simulink model "SanityCheckZ"  (R2023a)
settings: Solver=VariableStepAuto  StartTime=0.0  StopTime=10.0  RelTol=1e-3
settings Model: Creator=aan18022  LastModifiedBy=asd19005

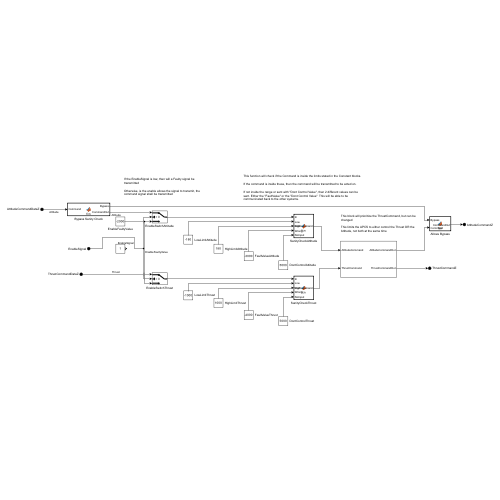
[thumbnail: Simulink's stored preview of the top-level diagram]
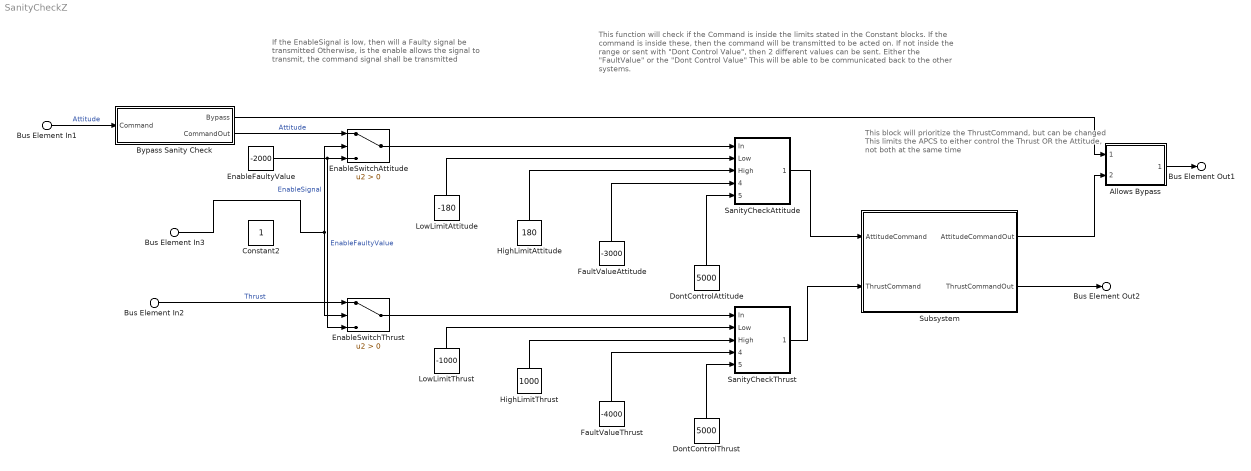
== system SanityCheckZ ==
  note: If the EnableSignal is low, then will a Faulty signal be transmitted
      |
      | Otherwise, is the enable allows the signal to transmit, the command signal shall be transmitted
  note: This function will check if the Command is inside the limits stated in the Constant blocks.
      |
      | If the command is inside these, then the command will be transmitted to be acted on.
      |
      | If not inside the range or sent with "Dont Control Value", then 2 different values can be sent. Either the "FaultValue" or the "Dont Control Value"  This will be able to be communicated back to the other systems.
  note: This block will prioritize the ThrustCommand, but can be changed
      |
      | This limits the APCS to either control the Thrust OR the Attitude, not both at the same time
  Bus Element In3 : Inport  PortName=EnableSignal
  Bus Element In1 : Inport  Port=2  PortName=AttitudeCommandDataZ
  Bus Element In2 : Inport  Port=3  PortName=ThrustCommandDataZ
  Allows Bypass : MATLAB Function  TreatAsAtomicUnit=on
  Bypass Sanity Check : MATLAB Function  TreatAsAtomicUnit=on
  Constant2 : Constant
  DontControlAttitude : Constant  Value=5000
  DontControlThrust : Constant  Value=5000
  EnableFaultyValue : Constant  Value=-2000
  EnableSwitchAttitude : Switch  Criteria=u2 > Threshold  SaturateOnIntegerOverflow=off  InputSameDT=off
  EnableSwitchThrust : Switch  Criteria=u2 > Threshold  SaturateOnIntegerOverflow=off  InputSameDT=off
  FaultValueAttitude : Constant  Value=-3000
  FaultValueThrust : Constant  Value=-4000
  HighLimitAttitude : Constant  Value=180
  HighLimitThrust : Constant  Value=1000
  LowLimitAttitude : Constant  Value=-180
  LowLimitThrust : Constant  Value=-1000
  SanityCheckAttitude : MATLAB Function  TreatAsAtomicUnit=on
  SanityCheckThrust : MATLAB Function  TreatAsAtomicUnit=on
  Subsystem : Subsystem
  Bus Element Out1 : Outport  PortName=AttitudeCommandZ
  Bus Element Out2 : Outport  Port=2  PortName=ThrustCommandZ
  wires:
  EnableSwitchThrust/1 -> SanityCheckThrust/1(In)
  FaultValueAttitude/1 -> SanityCheckAttitude/4(Wrong)
  EnableSwitchAttitude/1 -> SanityCheckAttitude/1(In)
  SanityCheckThrust/1(ThrustCommand) -> Subsystem/2(ThrustCommand)
  LowLimitAttitude/1 -> SanityCheckAttitude/2(Low)
  Bus Element In2/1 -> EnableSwitchThrust/1  "Thrust"
  SanityCheckAttitude/1(AttitudeCommand) -> Subsystem/1(AttitudeCommand)
  LowLimitThrust/1 -> SanityCheckThrust/2(Low)
  HighLimitThrust/1 -> SanityCheckThrust/3(High)
  FaultValueThrust/1 -> SanityCheckThrust/4(Wrong)
  Bus Element In1/1 -> Bypass Sanity Check/1(Command)  "Attitude"
  EnableFaultyValue/1 -> EnableSwitchAttitude/3, EnableSwitchThrust/3  "EnableFaultyValue"
  HighLimitAttitude/1 -> SanityCheckAttitude/3(High)
  DontControlThrust/1 -> SanityCheckThrust/5(NoInput)
  Bus Element In3/1 -> EnableSwitchAttitude/2, EnableSwitchThrust/2  "EnableSignal"
  DontControlAttitude/1 -> SanityCheckAttitude/5(NoInput)
  Subsystem/2(ThrustCommandOut) -> Bus Element Out2/1
  Bypass Sanity Check/2(CommandOut) -> EnableSwitchAttitude/1  "Attitude"
  Bypass Sanity Check/1(Bypass) -> Allows Bypass/1(Bypass)
  Allows Bypass/1(CommandOut) -> Bus Element Out1/1
  Subsystem/1(AttitudeCommandOut) -> Allows Bypass/2(Command)

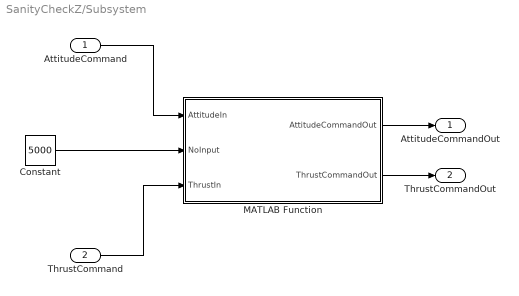
== system SanityCheckZ/Subsystem ==
  AttitudeCommand : Inport
  ThrustCommand : Inport  Port=2
  Constant : Constant  Value=5000
  MATLAB Function : MATLAB Function  TreatAsAtomicUnit=on
  AttitudeCommandOut : Outport
  ThrustCommandOut : Outport  Port=2
  wires:
  AttitudeCommand/1 -> MATLAB Function/1(AttitudeIn)
  ThrustCommand/1 -> MATLAB Function/3(ThrustIn)
  MATLAB Function/1(AttitudeCommandOut) -> AttitudeCommandOut/1
  MATLAB Function/2(ThrustCommandOut) -> ThrustCommandOut/1
  Constant/1 -> MATLAB Function/2(NoInput)

== matlab function SanityCheckZ/SanityCheckThrust ==
  data: In input; Out output; Low input; High input; Wrong input; NoInput input
function Out = fcn(In,Low,High,Wrong,NoInput)

if (In >=Low && In <= High)
    Out = In;
elseif In == NoInput
    Out = NoInput;
else
    Out = Wrong;
end

== matlab function SanityCheckZ/SanityCheckAttitude ==
  data: In input; Out output; Low input; High input; Wrong input; NoInput input
function Out = fcn(In,Low,High,Wrong,NoInput)

if (In >=Low && In <= High)
    Out = In;
elseif In == NoInput
    Out = NoInput;
else
    Out = Wrong;
end

== matlab function SanityCheckZ/Subsystem/MATLAB Function ==
  data: AttitudeIn input; NoInput input; AttitudeCommandOut output; ThrustIn input; ThrustCommandOut output
function [AttitudeCommandOut, ThrustCommandOut]= fcn(AttitudeIn, NoInput, ThrustIn)

if ThrustIn ~= NoInput
    ThrustCommandOut = ThrustIn;
    AttitudeCommandOut = NoInput;
else
    ThrustCommandOut = NoInput;
    AttitudeCommandOut = AttitudeIn;
end

== matlab function SanityCheckZ/Bypass Sanity Check ==
  data: Bypass output; Command input; CommandOut output
function [Bypass,CommandOut]= fcn(Command)

if Command >= 5820
    CommandOut = 5000;
    Bypass = Command;
else
    CommandOut = Command;
    Bypass = 0;
end

== matlab function SanityCheckZ/Allows Bypass ==
  data: Bypass input; CommandOut output; Command input
function CommandOut = fcn(Bypass,Command)

if Bypass ~=0
    CommandOut = Bypass-6000;
else
    CommandOut = Command;
end
